simulink model "carproject"  (R2016a)
settings: Solver=FixedStepAuto  StartTime=0.0  StopTime=inf  RelTol=1e-3
libraries: arduinolib x6
settings Model: SimulationMode=external  ExtModeTrigDuration=2  Creator=MOSTAFA  LastModifiedBy=MOSTAFA
settings OptimizationCC: OptimizeModelRefInitCode=on  LifeSpan=Inf  MaxStackSize=64
settings HardwareCC: ProdBitPerInt=16  ProdBitPerPointer=16  ProdLargestAtomicFloat=None  ProdWordSize=8  ProdHWDeviceType=Atmel->AVR
settings RTWCC: SystemTargetFile=ert.tlc  HardwareBoard=Arduino Uno  TemplateMakefile=ert_default_tmf  GenerateReport=on  Toolchain=Arduino AVR v1.6.1  BuildConfiguration=Faster Runs  IncludeHyperlinkInReport=on  LaunchReport=on  GenerateTraceInfo=on  GenerateTraceReport=on  GenerateTraceReportSl=on  GenerateTraceReportSf=on  GenerateTraceReportEml=on
settings CodeAppCC: ForceParamTrailComments=on  IgnoreCustomStorageClasses=off  OperatorAnnotations=on  SimulinkDataObjDesc=on  SFDataObjDesc=on  MATLABFcnDesc=on  InsertBlockDesc=on  MATLABSourceComments=on
settings ERTTargetCC: SupportContinuousTime=on  SupportVariableSizeSignals=on

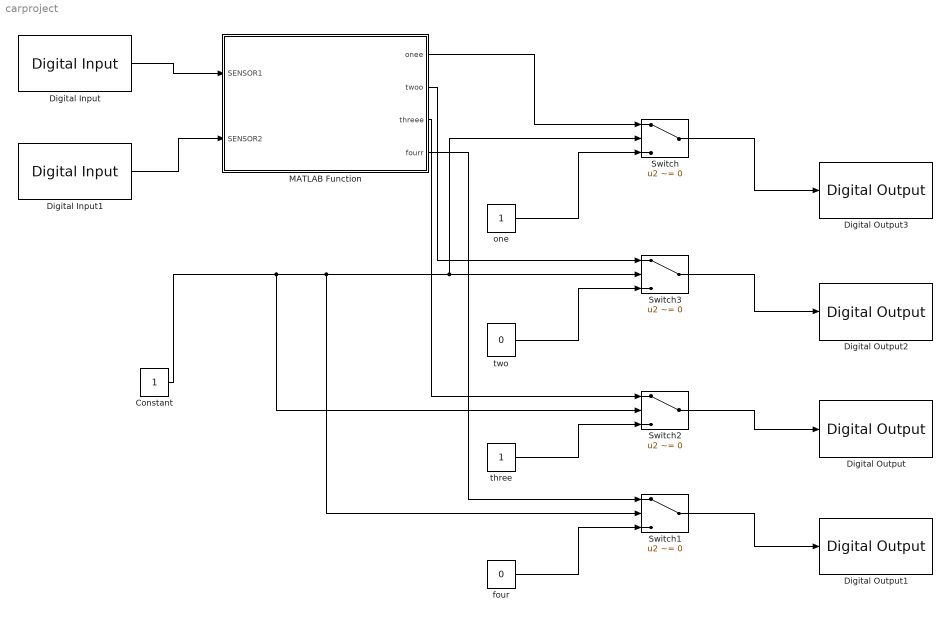
== system carproject ==
  Constant : Constant
  Digital Input : arduinolib/Digital Input  pinNumber=6  sampleTime=1  blockPlatform=arduino
  Digital Input1 : arduinolib/Digital Input  pinNumber=7  sampleTime=1  blockPlatform=arduino
  Digital Output : arduinolib/Digital Output  pinNumber=11  blockPlatform=arduino
  Digital Output1 : arduinolib/Digital Output  pinNumber=12  blockPlatform=arduino
  Digital Output2 : arduinolib/Digital Output  pinNumber=10  blockPlatform=arduino
  Digital Output3 : arduinolib/Digital Output  pinNumber=9  blockPlatform=arduino
  MATLAB Function : MATLAB Function  TreatAsAtomicUnit=on
  Switch{,1..3} (4 alike) : Switch  Criteria=u2 ~= 0
  four : Constant  Value=0
  one : Constant
  three : Constant
  two : Constant  Value=0
  wires:
  Digital Input/1 -> MATLAB Function/1(SENSOR1)
  Digital Input1/1 -> MATLAB Function/2(SENSOR2)
  MATLAB Function/1(onee) -> Switch/1
  one/1 -> Switch/3
  Constant/1 -> Switch2/2, Switch1/2, Switch3/2, Switch/2
  MATLAB Function/2(twoo) -> Switch3/1
  two/1 -> Switch3/3
  MATLAB Function/3(threee) -> Switch2/1
  three/1 -> Switch2/3
  MATLAB Function/4(fourr) -> Switch1/1
  four/1 -> Switch1/3
  Switch/1 -> Digital Output3/1
  Switch3/1 -> Digital Output2/1
  Switch2/1 -> Digital Output/1
  Switch1/1 -> Digital Output1/1

== matlab function carproject/MATLAB Function ==
  data: SENSOR1 input; onee output; SENSOR2 input; twoo output; threee output; fourr output
function [onee,twoo,threee,fourr] = fcn(SENSOR1,SENSOR2)
%#codegen

onee=0;
twoo=0;
threee=0;
fourr=0;
if(SENSOR1==1 && SENSOR2==1)
onee=1;
twoo=0;
threee=1;
fourr=0;
end
if(SENSOR1==1 && SENSOR2==0)
onee=1;
twoo=0;
threee=0;
fourr=0;
end
if(SENSOR1==0 && SENSOR2==1)
onee=0;
twoo=0;
threee=1;
fourr=0;
end
if(SENSOR1==0 && SENSOR2==0)
onee=0;
twoo=0;
threee=0;
fourr=0;
end
